simulink model "bpsk_rx_decim_cic"  (R2019a)
settings: Solver=VariableStepAuto  StartTime=0.0  StopTime=10000/64e6  RelTol=1e-3
InitFcn:
  | setup_bpsk_receiver
undefined symbols (not defined in the file): designMultirateFIR, tx_data, xlfda_numerator
libraries: xbsIndex_r4 x17, hdlsllib x11, dspmlti4 x9, dspswit3 x4, dspsigops x2, commrandsrc3 x1, simulink x1
(part 2 of 2)

== system bpsk_rx_decim_cic/BPSK System/BPSK TX Generation/DMA Read/Latch ==
  S : Inport
  R : Inport  Port=2
  Multiport Switch : MultiPortSwitch  DataPortOrder=Zero-based contiguous  Inputs=2  zeroidx=on
  Unit Delay Resettable Synchronous : hdlsllib/Discrete/Unit Delay Resettable Synchronous  InitialCondition=0.0  SampleTime=-1
      settings: SourceProductName=Simulink  SourceProductBaseCode=SL
  Q : Outport
  wires:
  Multiport Switch/1 -> Unit Delay Resettable Synchronous/1, Q/1
  S/1 -> Multiport Switch/3, Multiport Switch/1
  Unit Delay Resettable Synchronous/1 -> Multiport Switch/2
  R/1 -> Unit Delay Resettable Synchronous/2

== system bpsk_rx_decim_cic/BPSK System/BPSK TX Generation/DMA Read/Rising Edge Detector ==
  Input : Inport
  AND1 : Logic  IconShape=distinctive  AllPortsSameDT=off  OutDataTypeStr=boolean
  Delay1 : Delay  DelayLength=1
  NOT : Logic  Operator=NOT  IconShape=distinctive  AllPortsSameDT=off  OutDataTypeStr=boolean
  Output : Outport
  wires:
  NOT/1 -> AND1/1
  Input/1 -> AND1/2, Delay1/1
  Delay1/1 -> NOT/1
  AND1/1 -> Output/1

== system bpsk_rx_decim_cic/BPSK System/RF-ADC/NCO and Mixer/RF-ADC Coarse Mixer ==
  Data In : Inport
  Constant : Constant  Value=mc  OutDataTypeStr=fixdt(0,2,0)  SampleTime=-1
  Data Type Conversion : DataTypeConversion  OutDataTypeStr=fixdt(1,16,14)
  Multiport Switch1 : MultiPortSwitch  DataPortOrder=Zero-based contiguous  zeroidx=on
  Negate : Subsystem
  fs_2 : Subsystem
  fs_4 : Subsystem
  Data Out : Outport
  wires:
  Data Type Conversion/1 -> Data Out/1
  fs_4/1(Data Out) -> Multiport Switch1/3, Negate/1(Data In)
  Negate/1(Data Out) -> Multiport Switch1/4
  Data In/1 -> fs_2/1(Data In), fs_4/1(Data In)
  Constant/1 -> Multiport Switch1/1
  fs_2/1(Data Out) -> Multiport Switch1/2
  Multiport Switch1/1 -> Data Type Conversion/1

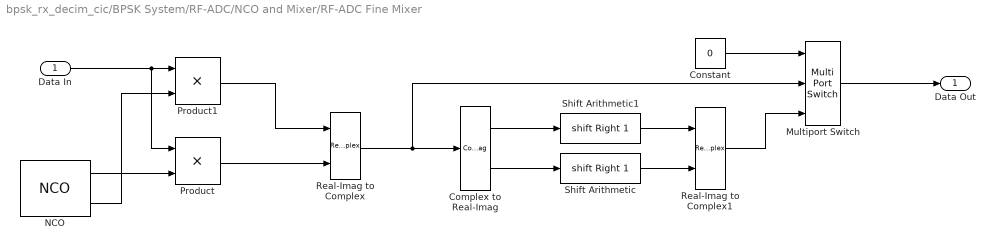
== system bpsk_rx_decim_cic/BPSK System/RF-ADC/NCO and Mixer/RF-ADC Fine Mixer ==
  Data In : Inport
  Complex to Real-Imag : ComplexToRealImag
  Constant : Constant  Value=0  SampleTime=-1
  Multiport Switch : MultiPortSwitch  DataPortOrder=Zero-based contiguous  Inputs=2  zeroidx=on
  NCO : dspsigops/NCO  AccIncSrc=Specify via dialog  AccInc=fix((((fc*1e9)*(2^18))/(fs))*2^30)  PhaseOffsetSrc=Specify via dialog  PhaseOffset=fix((((2^18)*fph)/(2*pi))*2^30)  AccumWL=48  HasDither=off  DitherWL=4  PNgeneratorLength=19  HasPhaseQuantizer=on  TableDepth=18  HasOutputPhaseError=off  Formula=Sine and cosine  DataType=Binary point scaling  OutputWL=16  OutputFL=14  CompMethod=Table lookup (no interpolation)  SampleTime=1/(fs)  SamplesPerFrame=ssr  OutputFrames=off
      settings: SourceProductName=DSP System Toolbox  SourceProductBaseCode=DS
  Product : Product  OutDataTypeStr=fixdt(1,16,14)
  Product1 : Product  OutDataTypeStr=fixdt(1,16,14)
  Real-Imag to Complex : RealImagToComplex
  Real-Imag to Complex1 : RealImagToComplex
  Shift Arithmetic : ArithShift  BitShiftNumber=1  BitShiftDirection=Right
  Shift Arithmetic1 : ArithShift  BitShiftNumber=1  BitShiftDirection=Right
  Data Out : Outport
  wires:
  Product/1 -> Real-Imag to Complex/2
  Product1/1 -> Real-Imag to Complex/1
  Real-Imag to Complex/1 -> Complex to Real-Imag/1, Multiport Switch/2
  NCO/2 -> Product1/2
  NCO/1 -> Product/2
  Real-Imag to Complex1/1 -> Multiport Switch/3
  Shift Arithmetic/1 -> Real-Imag to Complex1/2
  Shift Arithmetic1/1 -> Real-Imag to Complex1/1
  Complex to Real-Imag/1 -> Shift Arithmetic1/1
  Complex to Real-Imag/2 -> Shift Arithmetic/1
  Multiport Switch/1 -> Data Out/1
  Constant/1 -> Multiport Switch/1
  Data In/1 -> Product/1, Product1/1

== system bpsk_rx_decim_cic/BPSK System/RF-DAC/NCO and Mixer/RF-DAC Coarse Mixer ==
  Data In : Inport
  Add2 : Sum
  Complex to Real-Imag : ComplexToRealImag
  Constant : Constant  Value=mc  OutDataTypeStr=fixdt(0,2,0)  SampleTime=-1
  Multiport Switch1 : MultiPortSwitch  DataPortOrder=Zero-based contiguous  zeroidx=on
  Negate : Subsystem
  fs_2 : Subsystem
  fs_4 : Subsystem
  Data Out : Outport
  wires:
  Add2/1 -> Data Out/1
  Complex to Real-Imag/2 -> Add2/2
  Complex to Real-Imag/1 -> Add2/1
  Multiport Switch1/1 -> Complex to Real-Imag/1
  fs_2/1(Data Out) -> Multiport Switch1/2
  Constant/1 -> Multiport Switch1/1
  Data In/1 -> fs_4/1(Data In), fs_2/1(Data In)
  Negate/1(Data Out) -> Multiport Switch1/4
  fs_4/1(Data Out) -> Negate/1(Data In), Multiport Switch1/3

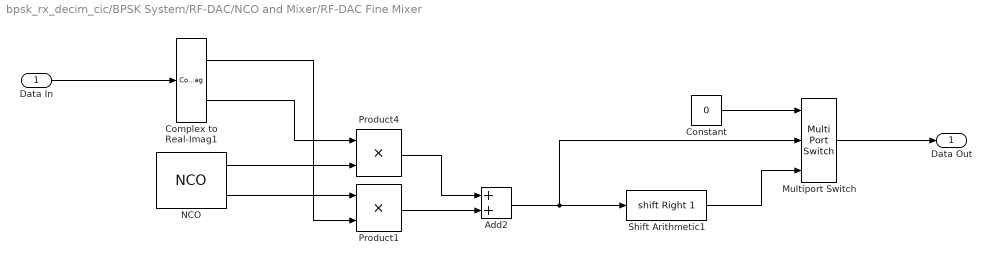
== system bpsk_rx_decim_cic/BPSK System/RF-DAC/NCO and Mixer/RF-DAC Fine Mixer ==
  Data In : Inport
  Add2 : Sum
  Complex to Real-Imag1 : ComplexToRealImag
  Constant : Constant  Value=0  OutDataTypeStr=boolean  SampleTime=-1
  Multiport Switch : MultiPortSwitch  DataPortOrder=Zero-based contiguous  Inputs=2  zeroidx=on
  NCO : dspsigops/NCO  AccIncSrc=Specify via dialog  AccInc=fix((((fc*1e9)*(2^18))/(fs))*2^30)  PhaseOffsetSrc=Specify via dialog  PhaseOffset=fix((((2^18)*fph)/(2*pi))*2^30)  AccumWL=48  HasDither=off  DitherWL=4  PNgeneratorLength=19  HasPhaseQuantizer=on  TableDepth=18  HasOutputPhaseError=off  Formula=Sine and cosine  DataType=Binary point scaling  OutputWL=16  OutputFL=14  CompMethod=Table lookup (no interpolation)  SampleTime=1/(fs)  SamplesPerFrame=ssr  OutputFrames=off
      settings: SourceProductName=DSP System Toolbox  SourceProductBaseCode=DS
  Product1 : Product  OutDataTypeStr=Inherit: Same as first input
  Product4 : Product  OutDataTypeStr=Inherit: Same as first input
  Shift Arithmetic1 : ArithShift  BitShiftNumber=1  BitShiftDirection=Right
  Data Out : Outport
  wires:
  Product1/1 -> Add2/2
  Complex to Real-Imag1/2 -> Product4/1
  Complex to Real-Imag1/1 -> Product1/2
  NCO/2 -> Product1/1
  NCO/1 -> Product4/2
  Product4/1 -> Add2/1
  Data In/1 -> Complex to Real-Imag1/1
  Constant/1 -> Multiport Switch/1
  Multiport Switch/1 -> Data Out/1
  Add2/1 -> Shift Arithmetic1/1, Multiport Switch/2
  Shift Arithmetic1/1 -> Multiport Switch/3

== system bpsk_rx_decim_cic/BPSK System/RF-ADC/NCO and Mixer/RF-ADC Coarse Mixer/Negate ==
  Data In : Inport
  Complex to Real-Imag2 : ComplexToRealImag
  Real-Imag to Complex1 : RealImagToComplex
  Unary Minus : UnaryMinus
  Data Out : Outport
  wires:
  Complex to Real-Imag2/1 -> Real-Imag to Complex1/1
  Real-Imag to Complex1/1 -> Data Out/1
  Data In/1 -> Complex to Real-Imag2/1
  Unary Minus/1 -> Real-Imag to Complex1/2
  Complex to Real-Imag2/2 -> Unary Minus/1

== system bpsk_rx_decim_cic/BPSK System/RF-ADC/NCO and Mixer/RF-ADC Coarse Mixer/fs_2 ==
  Data In : Inport
  Counter : dspswit3/Counter  Direction=Up  CountEvent=Free running  CounterSize=User defined  MaxCount=1  InitialCount=0  Output=Count  HitValue=32  ResetInput=off  SamplesPerFrame=ssr  Ts=1/(fs)  CntDtype=uint8  HitDtype=Logical
  Multiport Switch2 : MultiPortSwitch  DataPortOrder=Zero-based contiguous  Inputs=2  zeroidx=on
  Real-Imag to Complex : RealImagToComplex
  Real-Imag to Complex1 : RealImagToComplex
  Unary Minus1 : UnaryMinus
  Data Out : Outport
  wires:
  Unary Minus1/1 -> Real-Imag to Complex/1, Real-Imag to Complex/2
  Counter/1 -> Multiport Switch2/1
  Multiport Switch2/1 -> Data Out/1
  Real-Imag to Complex/1 -> Multiport Switch2/3
  Real-Imag to Complex1/1 -> Multiport Switch2/2
  Data In/1 -> Unary Minus1/1, Real-Imag to Complex1/2, Real-Imag to Complex1/1

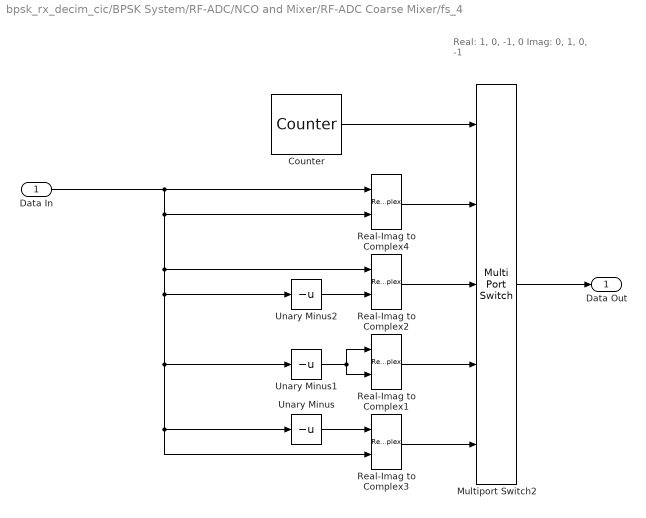
== system bpsk_rx_decim_cic/BPSK System/RF-ADC/NCO and Mixer/RF-ADC Coarse Mixer/fs_4 ==
  note: Real:	1, 0, -1, 0
      | Imag:	0, 1, 0, -1
  Data In : Inport
  Counter : dspswit3/Counter  Direction=Up  CountEvent=Free running  CounterSize=User defined  MaxCount=3  InitialCount=0  Output=Count  HitValue=32  ResetInput=off  SamplesPerFrame=ssr  Ts=1/(fs)  CntDtype=uint8  HitDtype=Logical
  Multiport Switch2 : MultiPortSwitch  DataPortOrder=Zero-based contiguous  Inputs=4  zeroidx=on
  Real-Imag to Complex{1..4} (4 alike) : RealImagToComplex
  Unary Minus : UnaryMinus
  Unary Minus1 : UnaryMinus
  Unary Minus2 : UnaryMinus
  Data Out : Outport
  wires:
  Multiport Switch2/1 -> Data Out/1
  Real-Imag to Complex3/1 -> Multiport Switch2/5
  Data In/1 -> Real-Imag to Complex4/2, Real-Imag to Complex2/1, Real-Imag to Complex3/2, Unary Minus/1, Unary Minus1/1, Unary Minus2/1, Real-Imag to Complex4/1
  Real-Imag to Complex2/1 -> Multiport Switch2/3
  Counter/1 -> Multiport Switch2/1
  Real-Imag to Complex1/1 -> Multiport Switch2/4
  Unary Minus1/1 -> Real-Imag to Complex1/1, Real-Imag to Complex1/2
  Real-Imag to Complex4/1 -> Multiport Switch2/2
  Unary Minus2/1 -> Real-Imag to Complex2/2
  Unary Minus/1 -> Real-Imag to Complex3/1

== system bpsk_rx_decim_cic/BPSK System/RF-DAC/NCO and Mixer/RF-DAC Coarse Mixer/Negate ==
  Data In : Inport
  Complex to Real-Imag2 : ComplexToRealImag
  Real-Imag to Complex1 : RealImagToComplex
  Unary Minus : UnaryMinus
  Data Out : Outport
  wires:
  Complex to Real-Imag2/2 -> Unary Minus/1
  Unary Minus/1 -> Real-Imag to Complex1/2
  Data In/1 -> Complex to Real-Imag2/1
  Real-Imag to Complex1/1 -> Data Out/1
  Complex to Real-Imag2/1 -> Real-Imag to Complex1/1

== system bpsk_rx_decim_cic/BPSK System/RF-DAC/NCO and Mixer/RF-DAC Coarse Mixer/fs_2 ==
  Data In : Inport
  Counter : dspswit3/Counter  Direction=Up  CountEvent=Free running  CounterSize=User defined  MaxCount=1  InitialCount=0  Output=Count  HitValue=32  ResetInput=off  SamplesPerFrame=ssr  Ts=1/(fs)  CntDtype=uint8  HitDtype=Logical
  Multiport Switch2 : MultiPortSwitch  DataPortOrder=Zero-based contiguous  Inputs=2  zeroidx=on
  Unary Minus : UnaryMinus
  Data Out : Outport
  wires:
  Data In/1 -> Unary Minus/1, Multiport Switch2/2
  Unary Minus/1 -> Multiport Switch2/3
  Counter/1 -> Multiport Switch2/1
  Multiport Switch2/1 -> Data Out/1

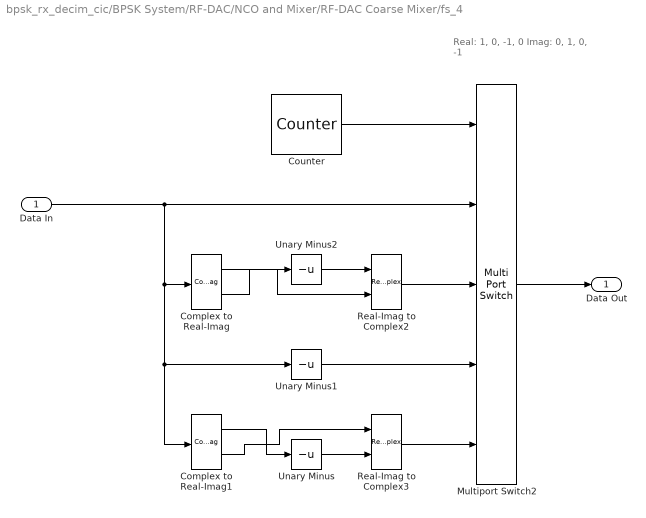
== system bpsk_rx_decim_cic/BPSK System/RF-DAC/NCO and Mixer/RF-DAC Coarse Mixer/fs_4 ==
  note: Real:	1, 0, -1, 0
      | Imag:	0, 1, 0, -1
  Data In : Inport
  Complex to Real-Imag : ComplexToRealImag
  Complex to Real-Imag1 : ComplexToRealImag
  Counter : dspswit3/Counter  Direction=Up  CountEvent=Free running  CounterSize=User defined  MaxCount=3  InitialCount=0  Output=Count  HitValue=32  ResetInput=off  SamplesPerFrame=ssr  Ts=1/(fs)  CntDtype=uint8  HitDtype=Logical
  Multiport Switch2 : MultiPortSwitch  DataPortOrder=Zero-based contiguous  Inputs=4  zeroidx=on
  Real-Imag to Complex2 : RealImagToComplex
  Real-Imag to Complex3 : RealImagToComplex
  Unary Minus : UnaryMinus
  Unary Minus1 : UnaryMinus
  Unary Minus2 : UnaryMinus
  Data Out : Outport
  wires:
  Counter/1 -> Multiport Switch2/1
  Real-Imag to Complex2/1 -> Multiport Switch2/3
  Complex to Real-Imag/1 -> Real-Imag to Complex2/2
  Unary Minus1/1 -> Multiport Switch2/4
  Data In/1 -> Unary Minus1/1, Complex to Real-Imag1/1, Complex to Real-Imag/1, Multiport Switch2/2
  Real-Imag to Complex3/1 -> Multiport Switch2/5
  Multiport Switch2/1 -> Data Out/1
  Complex to Real-Imag1/2 -> Real-Imag to Complex3/1
  Complex to Real-Imag1/1 -> Unary Minus/1
  Unary Minus/1 -> Real-Imag to Complex3/2
  Complex to Real-Imag/2 -> Unary Minus2/1
  Unary Minus2/1 -> Real-Imag to Complex2/1
